simulink model "simu_usv_step_ITPMC"  (R2022b)
settings: Solver=ode4  StartTime=0  StopTime=40  FixedStep=Ts_inner  RelTol=1e-3  EnableMultiTasking=on
InitFcn:
  | s=1;
StartFcn:
  | s=1;
values from neighbouring files (symbols this model uses):
  c = 0.02    [opt_USV_step2.m]    (also in setup_USV_ITPMC.m = 0.1)
  D = [4.5+sign(x(4))*1.32*x(4)+14.4*x(4)*x(4) 0 0 ... (first row only)    [opt_USV_step2.m]    (also in plant.m = [5.5+1.52*abs(x(4))+17.4*x(4)*x(4) 0 0; setup_USV_ITPMC.m)
  d1max = 10    [setup_USV_ITPMC.m]
  d2max = 0.5    [setup_USV_ITPMC.m]
  gamma1 = 10    [setup_USV_ITPMC.m]
  gamma2 = 10    [setup_USV_ITPMC.m]
  K1 = 10    [opt_USV_step2.m]    (also in setup_USV_ITPMC.m = 2)
  K2 = 10    [opt_USV_step2.m]    (also in setup_USV_ITPMC.m = 0.7)
  ks1 = 20    [setup_USV_ITPMC.m]
  ks2 = 9.5    [setup_USV_ITPMC.m]
  N = 100    [opt_USV_step2.m]    (also in setup_USV_ITPMC.m = 20)
  p1 = 50    [opt_USV_step2.m]    (also in setup_USV_ITPMC.m = 10)
  p2 = 50    [opt_USV_step2.m]    (also in setup_USV_ITPMC.m = 5)
  Ts_inner = 1e-1    (= 0.1)    [opt_USV_step2.m]    (also in setup_USV_ITPMC.m)
  uM1 = 120    [opt_USV_step2.m]    (also in setup_USV_ITPMC.m = 100)
  uM2 = 0    [opt_USV_step2.m]    (also in setup_USV_ITPMC.m)
  uM3 = 8    [opt_USV_step2.m]    (also in setup_USV_ITPMC.m = 6.6)
settings Model: Creator=LinYinjie  LastModifiedBy=Administrator
settings SolverCC: AlgebraicLoopSolver=LineSearch  AutoInsertRateTranBlk=on  InsertRTBMode=Always
settings DataIOCC: SaveFormat=StructureWithTime  ReturnWorkspaceOutputs=off
settings DebuggingCC: MultiTaskCondExecSysMsg=none  MultiTaskRateTransMsg=warning  UnconnectedInputMsg=warning  UnconnectedOutputMsg=warning  UnconnectedLineMsg=warning  SFMachineParentedDataDiag=warning  ArithmeticOperatorsInVariantConditions=warning
settings ModelReferenceCC: EnableRefExpFcnMdlSchedulingChecks=on
settings SFSimCC: CustomCodeUndefinedFunction=UseInterfaceOnly

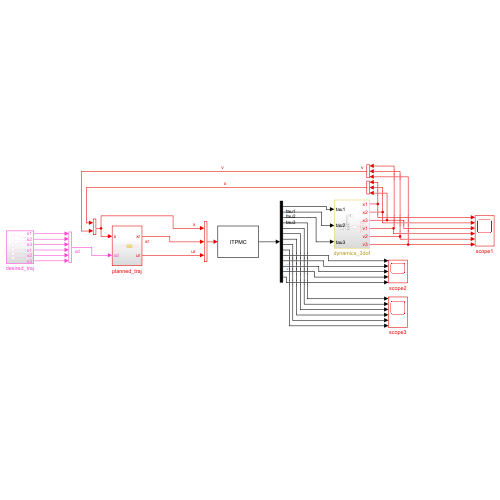
[thumbnail: Simulink's stored preview of the top-level diagram]
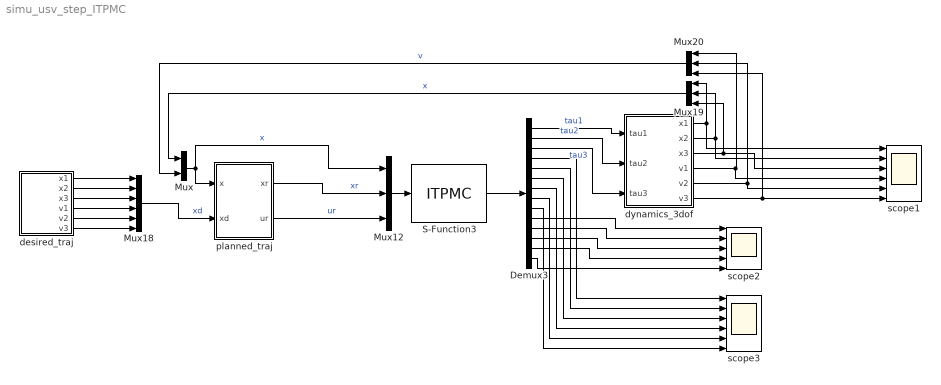
== system simu_usv_step_ITPMC ==
  Demux3 : Demux  Outputs=14
  Mux : Mux  Inputs=2
  Mux12 : Mux  Inputs=3
  Mux18 : Mux  Inputs=6
  Mux19 : Mux  Inputs=3
  Mux20 : Mux  Inputs=3
  S-Function3 : S-Function  FunctionName=ITPMC  Parameters=K1,K2,p1,p2,ks1,ks2,c,uM1,uM2,uM3,gamma1,gamma2,d1max,d2max,Ts_inner,N  SFunctionDeploymentMode=off  EnableBusSupport=off
  desired_traj : Subsystem
  dynamics_3dof : Subsystem
  planned_traj : Subsystem
  scope1 : Scope  NumInputPorts=6
  scope2 : Scope  NumInputPorts=5
  scope3 : Scope  NumInputPorts=6
  wires:
  Demux3/1 -> dynamics_3dof/1(tau1)  "tau1"
  Demux3/6 -> scope3/3
  Demux3/5 -> scope3/2
  Demux3/3 -> dynamics_3dof/3(tau3)  "tau3"
  Mux19/1 -> Mux/1  "x"
  Mux20/1 -> Mux/2  "v"
  Demux3/2 -> dynamics_3dof/2(tau2)  "tau2"
  Mux12/1 -> S-Function3/1
  S-Function3/1 -> Demux3/1
  Demux3/4 -> scope3/1
  planned_traj/2(ur) -> Mux12/3  "ur"
  Mux/1 -> planned_traj/1(x), Mux12/1  "x"
  Mux18/1 -> planned_traj/2(xd)  "xd"
  desired_traj/1(x1) -> Mux18/1
  desired_traj/6(v3) -> Mux18/6
  Demux3/7 -> scope3/4
  Demux3/8 -> scope3/5
  Demux3/9 -> scope3/6
  dynamics_3dof/1(x1) -> scope1/1, Mux19/1
  dynamics_3dof/2(x2) -> Mux19/2, scope1/2
  dynamics_3dof/3(x3) -> scope1/3, Mux19/3
  dynamics_3dof/4(v1) -> scope1/4, Mux20/1
  dynamics_3dof/5(v2) -> Mux20/2, scope1/5
  Demux3/10 -> scope2/1
  Demux3/11 -> scope2/2
  Demux3/12 -> scope2/3
  Demux3/13 -> scope2/4
  desired_traj/2(x2) -> Mux18/2
  desired_traj/3(x3) -> Mux18/3
  desired_traj/4(v1) -> Mux18/4
  desired_traj/5(v2) -> Mux18/5
  dynamics_3dof/6(v3) -> Mux20/3, scope1/6
  planned_traj/1(xr) -> Mux12/2  "xr"
  Demux3/14 -> scope2/5

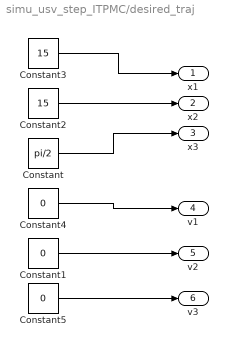
== system simu_usv_step_ITPMC/desired_traj ==
  Constant : Constant  Value=pi/2
  Constant1 : Constant  Value=0
  Constant2 : Constant  Value=15
  Constant3 : Constant  Value=15
  Constant4 : Constant  Value=0
  Constant5 : Constant  Value=0
  x1 : Outport
  x2 : Outport  Port=2
  x3 : Outport  Port=3
  v1 : Outport  Port=4
  v2 : Outport  Port=5
  v3 : Outport  Port=6
  wires:
  Constant1/1 -> v2/1
  Constant/1 -> x3/1
  Constant2/1 -> x2/1
  Constant3/1 -> x1/1
  Constant4/1 -> v1/1
  Constant5/1 -> v3/1

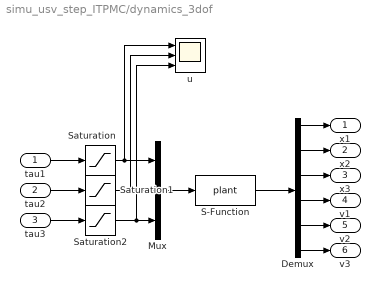
== system simu_usv_step_ITPMC/dynamics_3dof ==
  tau1 : Inport
  tau2 : Inport  Port=2
  tau3 : Inport  Port=3
  Demux : Demux  Outputs=6
  Mux : Mux  Inputs=3
  S-Function : S-Function  FunctionName=plant  Parameters=[0 0 -pi/4 0 0 0]  SFunctionDeploymentMode=off  EnableBusSupport=off
  Saturation : Saturate  UpperLimit=uM1  LowerLimit=0
  Saturation1 : Saturate  UpperLimit=uM2  LowerLimit=-uM2
  Saturation2 : Saturate  UpperLimit=uM3  LowerLimit=-uM3
  u : Scope  NumInputPorts=3
  x1 : Outport  VectorParamsAs1DForOutWhenUnconnected=off
  x2 : Outport  Port=2  VectorParamsAs1DForOutWhenUnconnected=off
  x3 : Outport  Port=3  VectorParamsAs1DForOutWhenUnconnected=off
  v1 : Outport  Port=4  VectorParamsAs1DForOutWhenUnconnected=off
  v2 : Outport  Port=5  VectorParamsAs1DForOutWhenUnconnected=off
  v3 : Outport  Port=6  VectorParamsAs1DForOutWhenUnconnected=off
  wires:
  tau1/1 -> Saturation/1
  Demux/1 -> x1/1
  Demux/4 -> v1/1
  tau2/1 -> Saturation1/1
  Demux/2 -> x2/1
  Demux/3 -> x3/1
  Saturation/1 -> u/1, Mux/1
  Saturation1/1 -> Mux/2, u/2
  S-Function/1 -> Demux/1
  Mux/1 -> S-Function/1
  tau3/1 -> Saturation2/1
  Saturation2/1 -> u/3, Mux/3
  Demux/5 -> v2/1
  Demux/6 -> v3/1

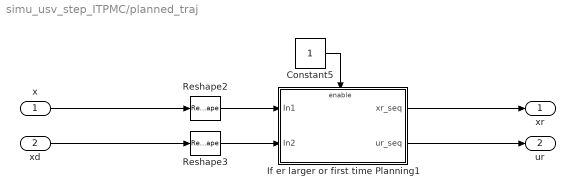
== system simu_usv_step_ITPMC/planned_traj ==
  x : Inport
  xd : Inport  Port=2
  Constant5 : Constant
  If er larger or first time Planning1 : Subsystem  TreatAsAtomicUnit=on
  Reshape2 : Reshape  OutputDimensionality=Column vector (2-D)
  Reshape3 : Reshape  OutputDimensionality=Column vector (2-D)
  xr : Outport
  ur : Outport  Port=2
  wires:
  xd/1 -> Reshape3/1
  x/1 -> Reshape2/1
  Reshape2/1 -> If er larger or first time Planning1/1(In1)
  Reshape3/1 -> If er larger or first time Planning1/2(In2)
  Constant5/1 -> If er larger or first time Planning1/Enable
  If er larger or first time Planning1/1(xr_seq) -> xr/1
  If er larger or first time Planning1/2(ur_seq) -> ur/1

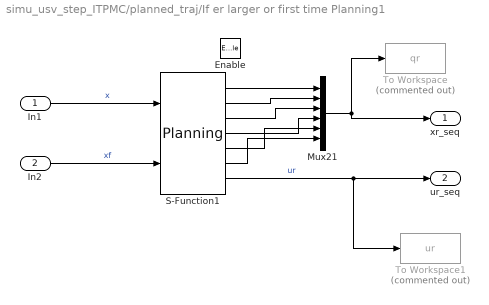
== system simu_usv_step_ITPMC/planned_traj/If er larger or first time Planning1 ==
  In1 : Inport
  In2 : Inport  Port=2
  Enable : EnablePort
  Mux21 : Mux  Inputs=6
  S-Function1 : S-Function  FunctionName=Planning  Parameters='Planning.casadi','Planning'  SFunctionDeploymentMode=off  EnableBusSupport=off
  To Workspace : ToWorkspace  Commented=on  VariableName=qr  SaveFormat=Structure With Time  SampleTime=-1
  To Workspace1 : ToWorkspace  Commented=on  VariableName=ur  SaveFormat=Structure With Time  SampleTime=-1
  xr_seq : Outport
  ur_seq : Outport  Port=2
  wires:
  S-Function1/7 -> ur_seq/1, To Workspace1/1  "ur"
  In1/1 -> S-Function1/1  "x"
  Mux21/1 -> xr_seq/1, To Workspace/1
  In2/1 -> S-Function1/2  "xf"
  S-Function1/1 -> Mux21/1
  S-Function1/2 -> Mux21/2
  S-Function1/3 -> Mux21/3
  S-Function1/4 -> Mux21/4
  S-Function1/5 -> Mux21/5
  S-Function1/6 -> Mux21/6
